simulink model "VehicleDynamics1Dof"  (R2025a)
settings: Solver=VariableStepAuto  StartTime=0.0  StopTime=10.0  RelTol=1e-3
undefined symbols (not defined in the file): d_transmission, M_vehicle
libraries: autolibshared x1
settings Model: DataDictionary=Vechicle1Dof.sldd  Creator=tecnicomcbti  LastModifiedBy=tecnicomcbti

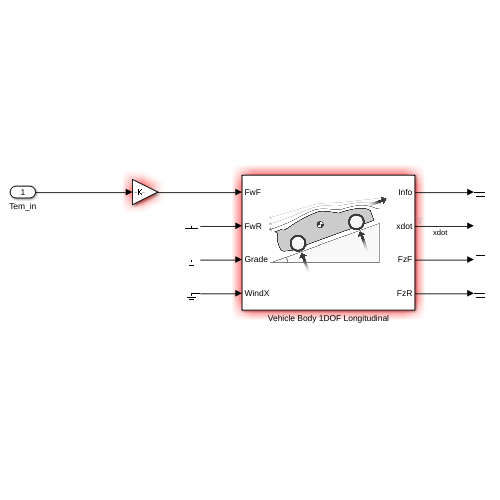
[thumbnail: Simulink's stored preview of the top-level diagram]
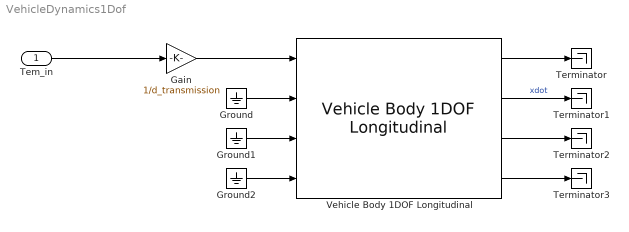
== system VehicleDynamics1Dof ==
  Tem_in : Inport
  Gain : Gain  Gain=1/d_transmission
  Ground : Ground
  Ground1 : Ground
  Ground2 : Ground
  Terminator{,1..3} (4 alike) : Terminator
  Vehicle Body 1DOF Longitudinal : autolibshared/Vehicle Body 1DOF Longitudinal  VariantControl=SL  extFMode=off  extMMode=off  extTamb=off  wind3D=off  aMode=2  NF=2  NR=2  m=M_vehicle  a=0.6  b=.8  h=.35  Cd=.3  Cl=0  Cpm=0  Af=Af_vehicle  x_o=0  xdot_o=0  Pabs=101325  T=273  g=9.81
      settings: LibrarySourceBlock=vehdynlibeom/Vehicle Body 1DOF Longitudinal
  wires:
  Ground/1 -> Vehicle Body 1DOF Longitudinal/2
  Ground1/1 -> Vehicle Body 1DOF Longitudinal/3
  Ground2/1 -> Vehicle Body 1DOF Longitudinal/4
  Vehicle Body 1DOF Longitudinal/1 -> Terminator/1
  Vehicle Body 1DOF Longitudinal/2 -> Terminator1/1  "xdot"
  Vehicle Body 1DOF Longitudinal/3 -> Terminator2/1
  Vehicle Body 1DOF Longitudinal/4 -> Terminator3/1
  Gain/1 -> Vehicle Body 1DOF Longitudinal/1
  Tem_in/1 -> Gain/1
